simulink model "ADCS_orbiter_detumbling"  (R2022a)
settings: Solver=ode4  StartTime=0.0  StopTime=21085  FixedStep=0.1  MaxStep=1  RelTol=1e-8
values from neighbouring files (symbols this model uses):
  A_cube = 1    [Data_detumbling.m]    (also in main_orbiter_detumbling.m = 12.9)
  A_S2B = [1,0,0;0,-1,0;0,0,-1]    [Data_detumbling.m]
  alpha_x = deg2rad(6/3600)    [Data_detumbling.m]
  alpha_y = deg2rad(6/3600)    [Data_detumbling.m]
  alpha_z = deg2rad(40/3600)    [Data_detumbling.m]
  B_ast = pinv(B)    [Data_detumbling.m]
  ceps = cos(eps)    [Data_detumbling.m]    (also in main_orbiter_detumbling.m)
  F_max = 0.650    (= 0.65)    [Data_detumbling.m]    (also in main_orbiter_detumbling.m = 1.13)
  F_min = 0.160    (= 0.16)    [Data_detumbling.m]    (also in main_orbiter_detumbling.m = 0.19)
  J = [Jx,0,0 ... (first row only)    [Data_detumbling.m]    (also in DisturbanceEvaluation.m = {J_NSO; J_SO}; Thruster_sizing_2.m = diag([12043.36, 15990.19, 8547.84]); main_orbiter.m = J_SO; main_orbiter_detumbling.m = J_SO)
  k_dx = G*J(1,1)/max(diag(J))    [main_orbiter_detumbling.m]
  k_dy = G*J(2,2)/max(diag(J))    [main_orbiter_detumbling.m]
  k_dz = G*J(3,3)/max(diag(J))    [main_orbiter_detumbling.m]
  k_p = 0    [Data_detumbling.m]    (also in main_orbiter_detumbling.m)
  n1 = [1;0;0]    [Data_detumbling.m]    (also in main_orbiter_detumbling.m)
  n2 = [0;1;0]    [Data_detumbling.m]    (also in main_orbiter_detumbling.m)
  n3 = [0;0;1]    [Data_detumbling.m]    (also in main_orbiter_detumbling.m)
  n4 = -n1    [Data_detumbling.m]    (also in main_orbiter_detumbling.m)
  n5 = -n2    [Data_detumbling.m]    (also in main_orbiter_detumbling.m)
  n6 = -n3    [Data_detumbling.m]    (also in main_orbiter_detumbling.m)
  n_sun = 2*pi/(365.25*24*3600)    (= 1.99102127766e-07)    [Data_detumbling.m]    (also in main_orbiter_detumbling.m)
  P = F_e/c    [Data_detumbling.m]    (also in main_orbiter_detumbling.m)
  qbn0 = qrand./norm(qrand)    [main_orbiter.m]    (also in main_orbiter_detumbling.m)
  R = diag([lx_mb/2 ly_mb/2 lz_mb/2]) * [0  0  1  1  0  0 -1 -1 ... (first row only)    [Data_detumbling.m]    (also in main_orbiter_detumbling.m = 0.5*[-ly*cos(inc)              ly*cos(inc)            ly*cos)
  R_ast = pinv(R)    [Data_detumbling.m]    (also in main_orbiter_detumbling.m)
  r_i = r_cube * [n1,n2,n3,n4,n5,n6]    [Data_detumbling.m]    (also in main_orbiter_detumbling.m = [lx/2-cm_off_x  -cm_off_x       -cm_off_x        lx/2+cm_off)
  rho_d = 0.1    [Data_detumbling.m]    (also in main_orbiter_detumbling.m)
  rho_s = 0.5    [Data_detumbling.m]    (also in main_orbiter_detumbling.m)
  S_star1 = S_star1/norm(S_star1)    [Data_detumbling.m]
  S_star2 = S_star2/norm(S_star2)    [Data_detumbling.m]
  S_star3 = S_star3/norm(S_star3)    [Data_detumbling.m]
  S_star4 = S_star4/norm(S_star4)    [Data_detumbling.m]
  seps = sin(eps)    [Data_detumbling.m]    (also in main_orbiter_detumbling.m)
  sigma_ARW = deg2rad(0.001)    [main_orbiter_detumbling.m]
  state0 = [r_vec_new; v_vec_new]    [main_orbiter_detumbling.m]
  w = ones(length(R(1,:)),1)    [Data_detumbling.m]    (also in main_orbiter_detumbling.m)
  w_c = [0 0 0]'    [Data_detumbling.m]    (also in main_orbiter_detumbling.m)
  wb0 = 0.0001*rand(3, 1)    [main_orbiter.m]    (also in main_orbiter_detumbling.m = 0.1*rand(3, 1))
libraries: vrlib x8, matrix_library x1, simulink x1
(part 3 of 3)

== system ADCS_orbiter_detumbling/Sensor and Attitude Determination/Subsystem3/Mapping choice/If Action Subsystem2/If Action Subsystem/If Action Subsystem1/From q3 ==
  A_I2B_err : Inport
  q3 : Inport  Port=2
  Divide : Product  Inputs=*/
  Divide1 : Product  Inputs=*/
  Divide2 : Product  Inputs=*/
  Gain9 : Gain  Gain=4
  Selector3 : Selector  NumberOfDimensions=2  InputPortWidth=3  IndexOptions=Index vector (dialog),Index vector (dialog)  Indices=1,3  OutputSizes=1,1
  Selector4 : Selector  NumberOfDimensions=2  InputPortWidth=3  IndexOptions=Index vector (dialog),Index vector (dialog)  Indices=3,1  OutputSizes=1,1
  Selector5 : Selector  NumberOfDimensions=2  InputPortWidth=3  IndexOptions=Index vector (dialog),Index vector (dialog)  Indices=3,2  OutputSizes=1,1
  Selector6 : Selector  NumberOfDimensions=2  InputPortWidth=3  IndexOptions=Index vector (dialog),Index vector (dialog)  Indices=2,3  OutputSizes=1,1
  Selector7 : Selector  NumberOfDimensions=2  InputPortWidth=3  IndexOptions=Index vector (dialog),Index vector (dialog)  Indices=1,2  OutputSizes=1,1
  Selector8 : Selector  NumberOfDimensions=2  InputPortWidth=3  IndexOptions=Index vector (dialog),Index vector (dialog)  Indices=2,1  OutputSizes=1,1
  Sum1 : Sum
  Sum2 : Sum
  Sum3 : Sum  Inputs=+-
  Vector Concatenate : Concatenate  NumInputs=4
  q_err : Outport
  wires:
  Divide/1 -> Vector Concatenate/4
  Divide1/1 -> Vector Concatenate/2
  Divide2/1 -> Vector Concatenate/1
  Selector7/1 -> Sum3/1
  Selector5/1 -> Sum2/1
  Selector3/1 -> Sum1/1
  Selector8/1 -> Sum3/2
  Sum2/1 -> Divide1/1  "q2"
  Vector Concatenate/1 -> q_err/1
  A_I2B_err/1 -> Selector7/1, Selector8/1, Selector3/1, Selector4/1, Selector5/1, Selector6/1
  Gain9/1 -> Divide/2, Divide1/2, Divide2/2
  Sum1/1 -> Divide2/1  "q1"
  q3/1 -> Gain9/1, Vector Concatenate/3  "q3"
  Selector4/1 -> Sum1/2
  Sum3/1 -> Divide/1  "q4"
  Selector6/1 -> Sum2/2

== matlab function ADCS_orbiter_detumbling/sample r, v/MATLAB Function ==
  data: t input; r output; A input; v output
function [r,v] = fcn(t, A)

t_ = floor(t+1);

if t_ >= 1
    r = A(1:3, t_);
    v = A(4:6, t_);
else
    r = A(1:3, 1);
    v = A(4:6, 1);
end
